simulink model "check_tiredata_lateral"  (R2018b)
settings: configuration reference "Physics" (kept outside this file)
undefined symbols (not defined in the file or in its folder): Aligning, Brakes, ContactPatch, Lateral, Longitudinal, omega0_Wheels_radps, Overturning, Rolling, Structural, TireSimulation, Turnslip, v0z_Wheels_mps, Vertical, Wheels, z0_TireDeflection_m
libraries: vehdynlibtire x1
settings Model: DataDictionary=check_tiredata.sldd  OrderedModelArguments=off  Creator=wischnewski  LastModifiedBy=ga25xiw

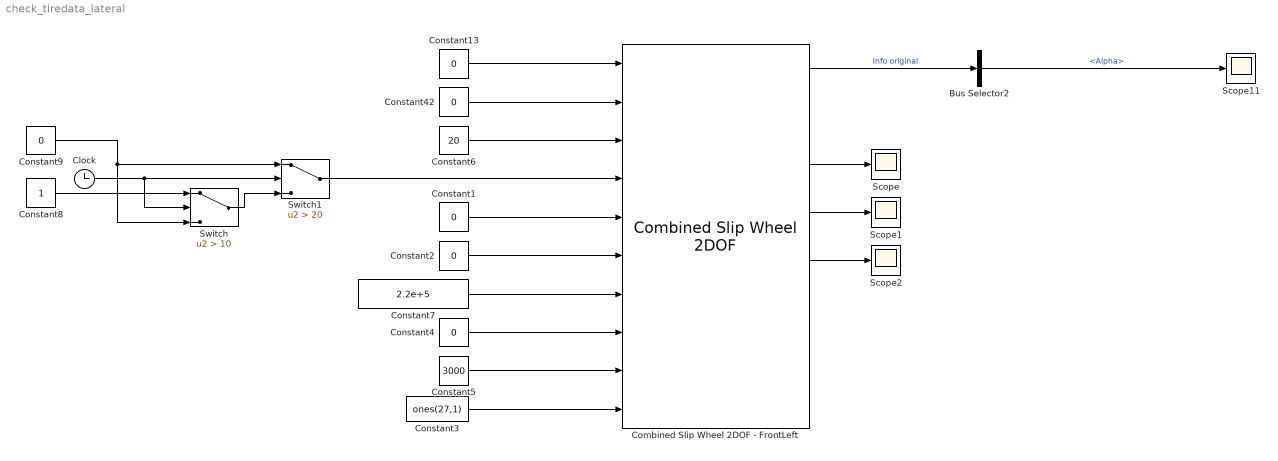
== system check_tiredata_lateral ==
  Bus Selector2 : BusSelector  OutputSignals=Alpha
  Clock : Clock
  Combined Slip Wheel 2DOF - FrontLeft : vehdynlibtire/Combined Slip Wheel 2DOF  BrakeType=Disc  mu_static=Brakes.mue_BrakePadsStaticFB (1)  mu_kinetic=Brakes.mue_BrakePadsKineticFB (1)  disk_abore=Brakes.d_BrakeBoreDiameterFB_m (1)  Rm=Brakes.r_BrakePadsMeanLeverRadiusFB_m (1)  num_pads=Brakes.n_BrakePadsNumberFB (1)  drum_abore=0.0508  drum_a=0.123  drum_c=0.212  drum_r=0.15  drum_theta1=0  drum_theta2=126  brake_p_bpt=[1 11.4736842105263 21.9473684210526 32.4210526315789 42.8947368421053 53.3684210526316 63.8421052631579 74.3157894736842 84.7894736842105 95.2631578947368 105.736842105263 116.210526315789 126.684210526316 137.157894736842 147.631578947368 158.105263157895 168.578947368421 179.052631578947 189.526315789474 200]  brake_n_bpt=[0 52.6315789473684 105.263157894737 157.894736842105 210.526315789474 263.157894736842 315.789473684211 368.421052631579 421.052631578947 473.684210526316 526.315789473684 578.947368421053 631.578947368421 684.210526315789 736.842105263158 789.473684210526 842.105263157895 894.736842105263 947.368421052632 1000]  f_brake_t=[43.4900602404453 42.5056030554862 41.5350898940194 40.5780454442085 39.6340111501808 38.7025443887544 37.7832176914519 36.8756180088306 35.9793460143796 35.0940154454303 34.2192524787115 33.3546951383474 32.4999927342521 31.6548053290159 30.8188032315107 29.991666515561 29.1730845621415 28.362755623661 27.5603864089927 26.765691687993;498.991217495636 487.695866636631 476.560505099801 465.579679307235 454.748127933653 444.060772460445 433.51270824929 423.099196101319 412.81565427025 402.657650900201 392.620896861006 382.701238955775 372.894653477208 363.197240090814 353.605216024701 344.114910546964 334.722759712992 325.425301366216 316.219170376863 307.10109410434;954.492374750826 932.886130217776 911.585920305583 890.581313170261 869.862244717126 849.419000532136 829.242198807128 809.322774193808 789.651962526121 770.221286354971 751.0225412433 732.047782773203 713.289314220164 694.739674852612 676.391628817892 658.238154578366 640.272434863842 622.48784710877 604.877954344734 587.436496520688;1409.99353200602 1378.07639379892 1346.61133551136 1315.58294703329 1284.9763615006 1254.77722860383 1224.97168936497 1195.5463522863 1166.48827078199 1137.78492180974 1109.42418562559 1081.39432659063 1053.68397496312 1026.28210961441 999.178041611083 972.361398609768 945.822110014692 919.550392851325 893.536738312604 867.771898937035;1865.49468926121 1823.26665738007 1781.63675071715 1740.58458089631 1700.09047828407 1660.13545667552 1620.7011799228 1581.76993037878 1543.32457903786 1505.34855726451 1467.82583000789 1430.74087040806 1394.07863570608 1357.82454437621 1321.96445440427 1286.48464264117 1251.37178516554 1216.61293859388 1182.19552228048 1148.10730135338;2320.9958465164 2268.45692096121 2216.66216592293 2165.58621475934 2115.20459506754 2065.49368474721 2016.43067048064 1967.99350847127 1920.16088729373 1872.91219271928 1826.22747439018 1780.08741422549 1734.47329644903 1689.36697913801 1644.75086719747 1600.60788667257 1556.92146031639 1513.67548433643 1470.85430624835 1428.44270376973;2776.49700377159 2713.64718454235 2651.68758112871 2590.58784862237 2530.31871185102 2470.8519128189 2412.16016103848 2354.21708656376 2296.9971955496 2240.47582817405 2184.62911877248 2129.43395804292 2074.86795719199 2020.9094138998 1967.53727999066 1914.73113070398 1862.47113546724 1810.73803007899 1759.51309021622 1708.77810618608;3231.99816102678 3158.8374481235 3086.71299633449 3015.58948248539 2945.43282863449 2876.21014089059 2807.88965159632 2740.44066465625 2673.83350380547 2608.03946362882 2543.03076315477 2478.78050186034 2415.26261793494 2352.4518486616 2290.32369278385 2228.85437473538 2168.02081061809 2107.80057582154 2048.17187418409 1989.11350860242;3687.49931828197 3604.02771170464 3521.73841154027 3440.59111634842 3360.54694541796 3281.56836896228 3203.61914215416 3126.66424274874 3050.66981206134 2975.60309908359 2901.43240753707 2828.12704567777 2755.6572786779 2683.9942834234 2613.11010557704 2542.97761876678 2473.57048576894 2404.8631215641 2336.83065815196 2269.44891101877;4143.00047553716 4049.21797528579 3956.76382674606 3865.59275021144 3775.66106220143 3686.92659703397 3599.34863271199 3512.88782084123 3427.50612031721 3343.16673453836 3259.83405191936 3177.4735894952 3096.05193942085 3015.5367181852 2935.89651837023 2857.10086279818 2779.12016091979 2701.92566730665 2625.48944211983 2549.78431343512;4598.50163279235 4494.40823886693 4391.78924195184 4290.59438407447 4190.77517898491 4092.28482510566 3995.07812326983 3899.11139893372 3804.34242857308 3710.73036999313 3618.23569630166 3526.82013331263 3436.44660016381 3347.079152947 3258.68293116342 3171.22410682959 3084.66983607064 2998.98821304921 2914.1482260877 2830.11971585147;5054.00279004754 4939.59850244808 4826.81465715762 4715.59601793749 4605.88929576838 4497.64305317735 4390.80761382767 4285.3349770262 4181.17873682896 4078.2940054479 3976.63734068395 3876.16667713006 3776.84126090677 3678.62158770879 3581.46934395661 3485.34735086099 ...(+2764 chars)]  tireParamSet=vdynPassCar.mat  plySteer=off  turnslip=off  PRESMAX=TireSimulation.PRESMAX(1)  PRESMIN=TireSimulation.PRESMIN(1)  FZMAX=TireSimulation.FZMAX(1)  FZMIN=TireSimulation.FZMIN(1)  VXLOW=TireSimulation.VXLOW(1)  KPUMAX=TireSimulation.KPUMAX(1)  KPUMIN=TireSimulation.KPUMIN(1)  ALPMAX=TireSimulation.ALPMAX(1)  ALPMIN=TireSimulation.ALPMIN(1)  CAMMAX=TireSimulation.CAMMAX(1)  CAMMIN=TireSimulation.CAMMIN(1)  LONGVL=TireSimulation.LONGVL(1)  omegao=omega0_Wheels_radps(1)  br=Wheels.mue_Wheels(1)  UNLOADED_RADIUS=Wheels.UNLOADED_RADIUS(1)  NOMPRES=Wheels.NOMPRES(1)  FNOMIN=Wheels.FNOMIN(1)  WIDTH=Wheels.WIDTH(1)  MASS=Wheels.m_WheelsFB_kg (1)  IYY=Wheels.Iyy_WheelsFB_kgm2 (1)  GRAVITY=- Wheels.a_Gravity_mps2  zo=z0_TireDeflection_m(1)  zdoto=v0z_Wheels_mps(1)  BREFF=Vertical.BREFF(1)  DREFF=Vertical.DREFF(1)  FREFF=Vertical.FREFF(1)  Q_RE0=Vertical.Q_RE0(1)  Q_V1=Vertical.Q_V1(1)  Q_V2=Vertical.Q_V2(1)  Q_FZ1=Vertical.Q_FZ1(1)  Q_FZ2=Vertical.Q_FZ2(1)  Q_FZ3=Vertical.Q_FZ3(1)  Q_FCX=Vertical.Q_FCX(1)  Q_FCY=Vertical.Q_FCY(1)  Q_FCY2=Vertical.Q_FCY2(1)  PFZ1=Vertical.PFZ1(1)  VERTICAL_STIFFNESS=Vertical.VERTICAL_STIFFNESS(1)  VERTICAL_DAMPING=Vertical.VERTICAL_DAMPING(1)  LONGITUDINAL_STIFFNESS=Structural.LONGITUDINAL_STIFFNESS(1)  LATERAL_STIFFNESS=Structural.LATERAL_STIFFNESS(1)  PCFX1=Structural.PCFX1(1)  PCFX2=Structural.PCFX2(1)  PCFX3=Structural.PCFX3(1)  PCFY1=Structural.PCFY1(1)  PCFY2=Structural.PCFY2(1)  PCFY3=Structural.PCFY3(1)  Q_RA1=ContactPatch.Q_RA1(1)  Q_RA2=ContactPatch.Q_RA2(1)  Q_RB1=ContactPatch.Q_RB1(1)  Q_RB2=ContactPatch.Q_RB2(1)  PCX1=Longitudinal.PCX1(1)  PDX1=Longitudinal.PDX1(1)  PDX2=Longitudinal.PDX2(1)  PDX3=Longitudinal.PDX3(1)  PEX1=Longitudinal.PEX1(1)  PEX2=Longitudinal.PEX2(1)  PEX3=Longitudinal.PEX3(1)  PEX4=Longitudinal.PEX4(1)  PKX1=Longitudinal.PKX1(1)  PKX2=Longitudinal.PKX2(1)  PKX3=Longitudinal.PKX3(1)  PHX1=Longitudinal.PHX1(1)  PHX2=Longitudinal.PHX2(1)  PVX1=Longitudinal.PVX1(1)  PVX2=Longitudinal.PVX2(1)  PPX1=Longitudinal.PPX1(1)  PPX2=Longitudinal.PPX2(1)  PPX3=Longitudinal.PPX3(1)  PPX4=Longitudinal.PPX4(1)  RBX1=Longitudinal.RBX1(1)  RBX2=Longitudinal.RBX2(1)  RBX3=Longitudinal.RBX3(1)  RCX1=Longitudinal.RCX1(1)  REX1=Longitudinal.REX1(1)  REX2=Longitudinal.REX2(1)  RHX1=Longitudinal.RHX1(1)  QSX1=Overturning.QSX1(1)  QSX2=Overturning.QSX2(1)  QSX3=Overturning.QSX3(1)  QSX4=Overturning.QSX4(1)  QSX5=Overturning.QSX5(1)  QSX6=Overturning.QSX6(1)  QSX7=Overturning.QSX7(1)  QSX8=Overturning.QSX8(1)  QSX9=Overturning.QSX9(1)  QSX10=Overturning.QSX10(1)  QSX11=Overturning.QSX11(1)  QSX12=Overturning.QSX12(1)  QSX13=Overturning.QSX13(1)  QSX14=Overturning.QSX14(1)  PPMX1=Overturning.PPMX1(1)  PCY1=Lateral.PCY1(1)  PDY1=Lateral.PDY1(1)  PDY2=Lateral.PDY2(1)  PDY3=Lateral.PDY3(1)  PEY1=Lateral.PEY1(1)  PEY2=Lateral.PEY2(1)  PEY3=Lateral.PEY3(1)  PEY4=Lateral.PEY4(1)  PEY5=Lateral.PEY5(1)  PKY1=Lateral.PKY1(1)  PKY2=Lateral.PKY2(1)  PKY3=Lateral.PKY3(1)  PKY4=Lateral.PKY4(1)  PKY5=Lateral.PKY5(1)  PKY6=Lateral.PKY6(1)  PKY7=Lateral.PKY7(1)  PHY1=Lateral.PHY1(1)  PHY2=Lateral.PHY2(1)  PVY1=Lateral.PVY1(1)  PVY2=Lateral.PVY2(1)  PVY3=Lateral.PVY3(1)  PVY4=Lateral.PVY4(1)  PPY1=Lateral.PPY1(1)  PPY2=Lateral.PPY2(1)  PPY3=Lateral.PPY3(1)  PPY4=Lateral.PPY4(1)  PPY5=Lateral.PPY5(1)  RBY1=Lateral.RBY1(1)  RBY2=Lateral.RBY2(1)  RBY3=Lateral.RBY3(1)  RBY4=Lateral.RBY4(1)  RCY1=Lateral.RCY1(1)  REY1=Lateral.REY1(1)  REY2=Lateral.REY2(1)  RHY1=Lateral.RHY1(1)  RHY2=Lateral.RHY2(1)  RVY1=Lateral.RVY1(1)  RVY2=Lateral.RVY2(1)  RVY3=Lateral.RVY3(1)  RVY4=Lateral.RVY4(1)  RVY5=Lateral.RVY5(1)  RVY6=Lateral.RVY6(1)  QSY1=Rolling.QSY1(1)  QSY2=Rolling.QSY2(1)  QSY3=Rolling.QSY3(1)  QSY4=Rolling.QSY4(1)  QSY5=Rolling.QSY5(1)  QSY6=Rolling.QSY6(1)  QSY7=Rolling.QSY7(1)  QSY8=Rolling.QSY8(1)  QBZ1=Aligning.QBZ1(1)  QBZ2=Aligning.QBZ2(1)  QBZ3=Aligning.QBZ3(1)  QBZ4=Aligning.QBZ4(1)  QBZ5=Aligning.QBZ5(1)  QBZ6=Aligning.QBZ6(1)  QBZ9=Aligning.QBZ9(1)  QBZ10=Aligning.QBZ10(1)  QCZ1=Aligning.QCZ1(1)  QDZ1=Aligning.QDZ1(1)  QDZ2=Aligning.QDZ2(1)  QDZ3=Aligning.QDZ3(1)  QDZ4=Aligning.QDZ4(1)  QDZ6=Aligning.QDZ6(1)  QDZ7=Aligning.QDZ7(1)  QDZ8=Aligning.QDZ8(1)  QDZ9=Aligning.QDZ9(1)  QDZ10=Aligning.QDZ10(1)  QDZ11=Aligning.QDZ11(1)  QEZ1=Aligning.QEZ1(1)  QEZ2=Aligning.QEZ2(1)  QEZ3=Aligning.QEZ3(1)  QEZ4=Aligning.QEZ4(1)  QEZ5=Aligning.QEZ5(1)  QHZ1=Aligning.QHZ1(1)  QHZ2=Aligning.QHZ2(1)  QHZ3=Aligning.QHZ3(1)  QHZ4=Aligning.QHZ4(1)  PPZ1=Aligning.PPZ1(1)  PPZ2=Aligning.PPZ2(1)  SSZ1=Aligning.SSZ1(1)  SSZ2=Aligning.SSZ2(1)  SSZ3=Aligning.SSZ3(1)  SSZ4=Aligning.SSZ4(1)  PDXP1=Turnslip.PDXP1(1)  PDXP2=Turnslip.PDXP2(1)  PDXP3=Turnslip.PDXP3(1)  PKYP1=Turnslip.PKYP1(1)  PDYP1=Turnslip.PDYP1(1)  PDYP2=Turnslip.PDYP2(1)  PDYP3=Turnslip.PDYP3(1)  PDYP4=Turnslip.PDYP4(1)  PHYP1=Turnslip.PHYP1(1)  PHYP2=Turnslip.PHYP2(1)  PHYP3=Turnslip.PHYP3(1)  PHYP4=Turnslip.PHYP4(1)  PECP1=Turnslip.PECP1(1)  PECP2=Turnslip.PECP2(1)  QDTP1=Turnslip.QDTP1(1)  QCRP1=Turnslip.QCRP1(1)  QCRP2=Turnslip.QCRP2(1)  QBRP1=Turnslip.QBRP1(1)  QDRP1=Turnslip.QDRP1(1)  QDRP2=Turnslip.QDRP2(1)  aMode=2
      settings: SourceProductName=Vehicle Dynamics Blockset  SourceProductBaseCode=VE
  Constant{1..2,4,9,13,42} (6 alike) : Constant  Value=0
  Constant3 : Constant  Value=ones(27,1)
  Constant5 : Constant  Value=3000
  Constant6 : Constant  Value=20
  Constant7 : Constant  Value=2.2e+5
  Constant8 : Constant
  Scope{,1..2,11} (4 alike) : Scope
  Switch : Switch  Criteria=u2 > Threshold  Threshold=10
  Switch1 : Switch  Criteria=u2 > Threshold  Threshold=20
  wires:
  Constant13/1 -> Combined Slip Wheel 2DOF - FrontLeft/1
  Constant3/1 -> Combined Slip Wheel 2DOF - FrontLeft/10
  Constant5/1 -> Combined Slip Wheel 2DOF - FrontLeft/9
  Constant4/1 -> Combined Slip Wheel 2DOF - FrontLeft/8
  Constant7/1 -> Combined Slip Wheel 2DOF - FrontLeft/7
  Constant2/1 -> Combined Slip Wheel 2DOF - FrontLeft/6
  Constant1/1 -> Combined Slip Wheel 2DOF - FrontLeft/5
  Combined Slip Wheel 2DOF - FrontLeft/3 -> Scope/1
  Combined Slip Wheel 2DOF - FrontLeft/4 -> Scope1/1
  Combined Slip Wheel 2DOF - FrontLeft/5 -> Scope2/1
  Bus Selector2/1 -> Scope11/1  "<Alpha>"
  Combined Slip Wheel 2DOF - FrontLeft/1 -> Bus Selector2/1  "Info original"
  Constant6/1 -> Combined Slip Wheel 2DOF - FrontLeft/3
  Switch1/1 -> Combined Slip Wheel 2DOF - FrontLeft/4
  Constant9/1 -> Switch/3, Switch1/1
  Constant8/1 -> Switch/1
  Clock/1 -> Switch1/2, Switch/2
  Switch/1 -> Switch1/3
  Constant42/1 -> Combined Slip Wheel 2DOF - FrontLeft/2
